simulink model "punto3"  (R2024a)
settings: Solver=ode4  StartTime=0.0  StopTime=10.0  FixedStep=0.003  RelTol=1e-3
settings Model: Creator=Usuario  LastModifiedBy=Usuario

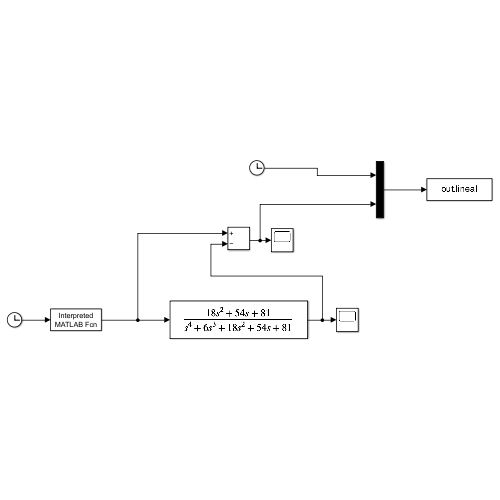
[thumbnail: Simulink's stored preview of the top-level diagram]
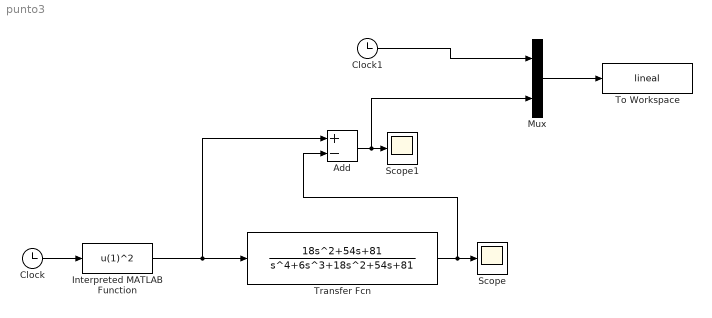
== system punto3 ==
  Add : Sum  Inputs=+-
  Clock : Clock
  Clock1 : Clock
  Interpreted MATLAB Function : MATLABFcn  MATLABFcn=u(1)^2
  Mux : Mux  Inputs=2
  Scope : Scope
  Scope1 : Scope
  To Workspace : ToWorkspace  VariableName=lineal  SampleTime=-1
  Transfer Fcn : TransferFcn  Numerator=[18 54 81]  Denominator=[1 6 18 54 81]
  wires:
  Clock/1 -> Interpreted MATLAB Function/1
  Interpreted MATLAB Function/1 -> Add/1, Transfer Fcn/1
  Transfer Fcn/1 -> Scope/1, Add/2
  Add/1 -> Mux/2, Scope1/1
  Mux/1 -> To Workspace/1
  Clock1/1 -> Mux/1
